simulink model "BIPVT_FullSystem"  (R2024b)
settings: Solver=VariableStepAuto  StartTime=0.0  StopTime=8760  RelTol=1e-3
PreLoadFcn:
  | % Pre-load all input data for BIPVT system
  | run('Load_Beckley_ThermalDemand.m');
  | run('generate_ElectricLoad.m');
libraries: spspowerguiLib x1

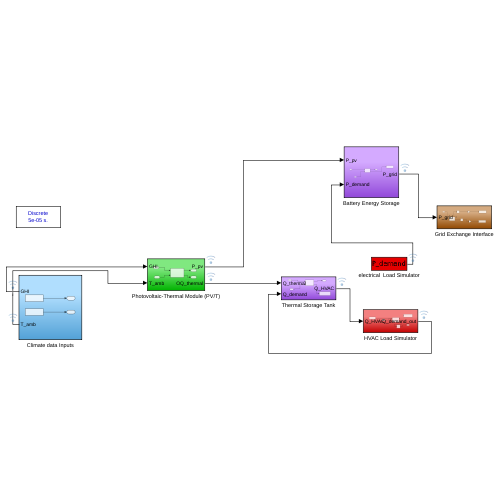
[thumbnail: Simulink's stored preview of the top-level diagram]
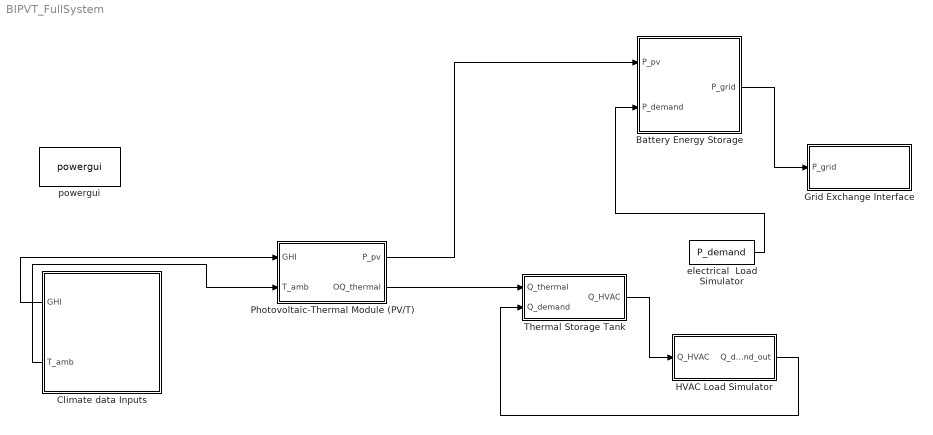
== system BIPVT_FullSystem ==
  Battery Energy Storage : Subsystem
  Climate data Inputs : Subsystem
  Grid Exchange Interface : Subsystem
  HVAC Load Simulator : Subsystem
  Photovoltaic-Thermal Module (PV/T) : Subsystem
  "Thermal Storage Tank " : Subsystem
  electrical  Load Simulator : FromWorkspace  VariableName=P_demand
  powergui : spspowerguiLib/powergui  Priority=1  SimulationMode=Discrete  SampleTime=50e-6  frequency=60  Iterations=50  frequencyindice=60  Pbase=100e6  ErrMax=1e-4  UnitsV=kV  UnitsW=MW  buscounter=0  FunctionMessages=off  echomessages=off  EnableUseOfTLC=off  CurrentSourceSwitches=off  DisableSnubberDevices=off  DisableRonSwitches=off  DisableVfSwitches=off  DisplayEquations=off  AutomaticDiscreteSolvers=off  SolverType=Tustin/Backward Euler (TBE)  Interpol=off  ExternalGateDelay=off  methode=off  Ts=100  x0status=blocks  SPID=on  SwTol=0  HookPort=off  NonlinearTolerance=1e-4  nMaxIteration=100  ContinueOnMaxIteration=off  RestoreLinks=warning  ResistiveCurrentMeasurement=off  Frange=[0:2:500]  Ylog=off  Xlog=on  ShowGrid=off  save=off  variable=ZData  structure=0  ZoomFFT=off  StartTime=0.0  cycles=1  DisplayStyle=1  fundamental=60  FreqAxis=off  MaxFrequency=1000  frequencyindicesteady=1  RmsSteady=1  display=off
  wires:
  Photovoltaic-Thermal Module (PV/T)/2(OQ_thermal) -> "Thermal Storage Tank "/1(Q_thermal)
  "Thermal Storage Tank "/1(Q_HVAC) -> HVAC Load Simulator/1(Q_HVAC)
  HVAC Load Simulator/1(Q_demand_out) -> "Thermal Storage Tank "/2(Q_demand)
  Photovoltaic-Thermal Module (PV/T)/1(P_pv) -> Battery Energy Storage/1(P_pv)
  Battery Energy Storage/1(P_grid) -> Grid Exchange Interface/1("P_grid ")
  electrical  Load Simulator/1 -> Battery Energy Storage/2(P_demand)
  Climate data Inputs/1(GHI) -> Photovoltaic-Thermal Module (PV/T)/1(GHI)
  Climate data Inputs/2(T_amb) -> Photovoltaic-Thermal Module (PV/T)/2(T_amb)

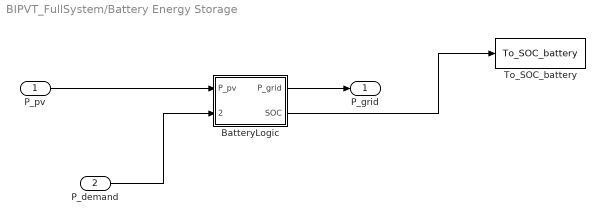
== system BIPVT_FullSystem/Battery Energy Storage ==
  P_pv : Inport
  P_demand : Inport  Port=2
  "BatteryLogic " : MATLAB Function  TreatAsAtomicUnit=on
  To_SOC_battery : ToWorkspace  VariableName=To_SOC_battery  SaveFormat=Timeseries  SampleTime=-1
  P_grid : Outport
  wires:
  P_pv/1 -> "BatteryLogic "/1(P_pv)
  P_demand/1 -> "BatteryLogic "/2(P_demand)
  "BatteryLogic "/1(P_grid) -> P_grid/1
  "BatteryLogic "/2(SOC) -> To_SOC_battery/1

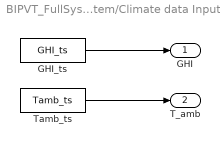
== system BIPVT_FullSystem/Climate data Inputs ==
  GHI_ts : FromWorkspace  VariableName=GHI_ts
  Tamb_ts : FromWorkspace  VariableName=Tamb_ts
  GHI : Outport
  T_amb : Outport  Port=2
  wires:
  GHI_ts/1 -> GHI/1
  Tamb_ts/1 -> T_amb/1

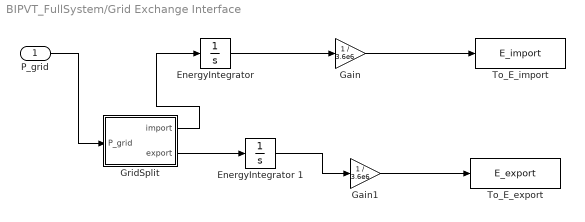
== system BIPVT_FullSystem/Grid Exchange Interface ==
  "P_grid " : Inport
  "EnergyIntegrator " : Integrator
  EnergyIntegrator 1 : Integrator
  Gain : Gain  Gain=1 / 3.6e6
  Gain1 : Gain  Gain=1 / 3.6e6
  GridSplit : MATLAB Function  TreatAsAtomicUnit=on
  To_E_export : ToWorkspace  VariableName=E_export  SaveFormat=Timeseries  SampleTime=-1
  To_E_import : ToWorkspace  VariableName=E_import  SaveFormat=Timeseries  SampleTime=-1
  wires:
  "EnergyIntegrator "/1 -> Gain/1
  "P_grid "/1 -> GridSplit/1(P_grid)
  GridSplit/1(import) -> "EnergyIntegrator "/1
  GridSplit/2(export) -> EnergyIntegrator 1/1
  EnergyIntegrator 1/1 -> Gain1/1
  Gain/1 -> To_E_import/1
  Gain1/1 -> To_E_export/1

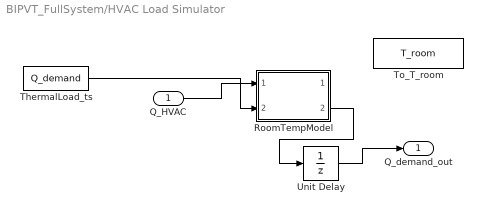
== system BIPVT_FullSystem/HVAC Load Simulator ==
  Q_HVAC : Inport
  RoomTempModel : MATLAB Function  TreatAsAtomicUnit=on
  ThermalLoad_ts : FromWorkspace  VariableName=Q_demand
  To_T_room : ToWorkspace  VariableName=T_room  SaveFormat=Timeseries  SampleTime=-1
  Unit Delay : UnitDelay  SampleTime=-1  HasFrameUpgradeWarning=on
  Q_demand_out : Outport
  wires:
  Q_HVAC/1 -> RoomTempModel/1(Q_HVAC)
  ThermalLoad_ts/1 -> RoomTempModel/2(Q_demand)
  RoomTempModel/2(Q_demand_out) -> Unit Delay/1
  Unit Delay/1 -> Q_demand_out/1

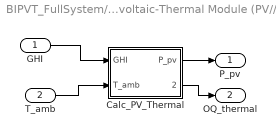
== system BIPVT_FullSystem/Photovoltaic-Thermal Module (PV//T) ==
  GHI : Inport
  T_amb : Inport  Port=2
  "Calc_PV_Thermal " : MATLAB Function  TreatAsAtomicUnit=on
  P_pv : Outport
  OQ_thermal : Outport  Port=2
  wires:
  GHI/1 -> "Calc_PV_Thermal "/1(GHI)
  T_amb/1 -> "Calc_PV_Thermal "/2(T_amb)
  "Calc_PV_Thermal "/1(P_pv) -> P_pv/1
  "Calc_PV_Thermal "/2(Q_thermal) -> OQ_thermal/1

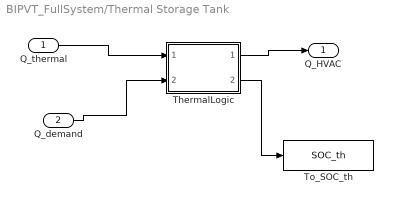
== system BIPVT_FullSystem/Thermal Storage Tank  ==
  Q_thermal : Inport
  Q_demand : Inport  Port=2
  "ThermalLogic " : MATLAB Function  TreatAsAtomicUnit=on
  To_SOC_th : ToWorkspace  VariableName=SOC_th  SaveFormat=Timeseries  SampleTime=-1
  Q_HVAC : Outport
  wires:
  Q_thermal/1 -> "ThermalLogic "/1(Q_thermal)
  "ThermalLogic "/1(Q_HVAC) -> Q_HVAC/1
  Q_demand/1 -> "ThermalLogic "/2(Q_demand)
  "ThermalLogic "/2(SOC_th) -> To_SOC_th/1

== matlab function BIPVT_FullSystem/Photovoltaic-Thermal Module (PV//T)/Calc_PV_Thermal  ==
  data: GHI input; P_pv output; T_amb input; Q_thermal output
function [P_pv, Q_thermal] = Calc_PV_Thermal_vec(GHI, T_amb)
    %GHI and T_amb can be scalars or vectors of the same length
    
    area   = 115;     % m² total PV area
    eta_pv = 0.16;    % panel efficiency
    derate = 0.85;    % system derating factor
    beta   = 0.0045;  % temperature coefficient (absolute value)
    refT   = 25;      % reference temperature (°C)
    
    % Electrical power (vectorized)
    P_ideal = GHI .* eta_pv .* area .* derate;
    tempFactor = 1 - beta .* (T_amb - refT);
    P_pv = P_ideal .* tempFactor;
    
    % Clip negatives to zero
    P_pv = max(P_pv, 0);
    
    % Thermal output (50% of remaining solar)
    Q_thermal = GHI .* 0.50 .* area .* derate;
end

== matlab function BIPVT_FullSystem/Thermal Storage Tank /ThermalLogic  ==
  settings: updateMethod=DISCRETE
  data: Q_thermal input; Q_HVAC output; Q_demand input; SOC_th output
function [Q_HVAC, SOC_th] = ThermalLogic(Q_thermal, Q_demand)
% ThermalLogic
% Manages charge/discharge of a hot water tank based on solar thermal input
% and actual room demand from HVAC_Load.

% Inputs:
%   Q_thermal - thermal energy input from PV/T module [W]
%   Q_demand  - thermal load requested by HVAC_Load subsystem [W]
%
% Outputs:
%   Q_HVAC    - thermal energy delivered to HVAC [W]
%   SOC_th    - current thermal energy stored [kWh]

    persistent soc
    if isempty(soc)
        soc = 5;  % Initial tank SOC [kWh]
    end

    cap = 10;  % Max tank capacity [kWh]

    % Convert both to kWh for internal consistency
    Q_thermal_kWh = Q_thermal / 1000;
    Q_demand_kWh = Q_demand / 1000;

    % Charge if solar energy is available
    if Q_thermal_kWh > 0
        charge = min(Q_thermal_kWh, cap - soc);
        soc = soc + charge;
    end

    % Deliver heat based on current SOC
    discharge = min(soc, Q_demand_kWh);
    soc = soc - discharge;

    % Convert output back to W
    Q_HVAC = discharge * 1000;
    SOC_th = soc;
end

== matlab function BIPVT_FullSystem/HVAC Load Simulator/RoomTempModel ==
  settings: updateMethod=DISCRETE
  data: Q_HVAC input; T_room output; Q_demand_out output; Q_demand input
function [T_room, Q_demand_out] = RoomModel(Q_HVAC, Q_demand)
    persistent T
    if isempty(T)
        T = 18;  % Initial room temp (°C)
    end

    % Room thermal properties
    V = 40;  % m³
    rho = 1.2;  % kg/m³
    c_p = 1005; % J/kg·K
    C_th = V * rho * c_p / 3600; % Wh/°C

    T_out = 5;     % Outside temp (°C)
    U = 0.9;       % W/°C loss
    dt = 1;        % seconds

    Q_loss = U * (T - T_out);
    dT = (Q_HVAC - Q_loss) * dt / C_th;
    T = T + dT;

    T_room = T;
    Q_demand_out = Q_demand;
end

== matlab function BIPVT_FullSystem/Grid Exchange Interface/GridSplit ==
  data: P_grid input; import output; export output
function [import, export] = GridSplit(P_grid)
    if P_grid > 0
        import = P_grid;
        export = 0;
    else
        import = 0;
        export = -P_grid; % make positive
    end
end

== matlab function BIPVT_FullSystem/Battery Energy Storage/BatteryLogic  ==
  settings: updateMethod=DISCRETE
  data: P_pv input; P_grid output; SOC output; P_demand input
function [P_grid, SOC] = BatteryLogic(P_pv, P_demand)
% BatteryLogic - Simulates charge/discharge of a battery system
% Inputs:
%   P_pv      - Power generated by PV (Watts)
%   P_demand  - Building electric load demand (Watts)
% Outputs:
%   P_grid    - Net power exchanged with the grid (Watts)
%   SOC       - Battery state of charge (kWh)

    persistent soc
    if isempty(soc)
        soc = 10;  % Initial SOC in kWh
    end

    capacity = 20;   % Battery capacity in kWh
    eff = 0.95;      % Round-trip efficiency

    % Power surplus or deficit
    surplus = P_pv - P_demand;

    % Convert power to energy per time step (assuming 1s step)
    deltaE = abs(surplus) / 1000;  % convert W to kWh for 1-second step

    if surplus > 0
        % Charging
        charge = min(deltaE * eff, capacity - soc);
        soc = soc + charge;
        P_grid = surplus - (charge / eff * 1000);  % back to W
    else
        % Discharging
        draw = min(deltaE / eff, soc);
        soc = soc - draw;
        P_grid = -(abs(surplus) - draw * eff * 1000);  % back to W
    end

    SOC = soc;
end
